simulink model "sampleModel386_pp_100_1"  (R2021b)
settings: Solver=VariableStepAuto  StartTime=0.0  StopTime=10.0  RelTol=1e-3
libraries: simulink x2, slpidlib x1
settings Model: Creator=user  LastModifiedBy=cemery

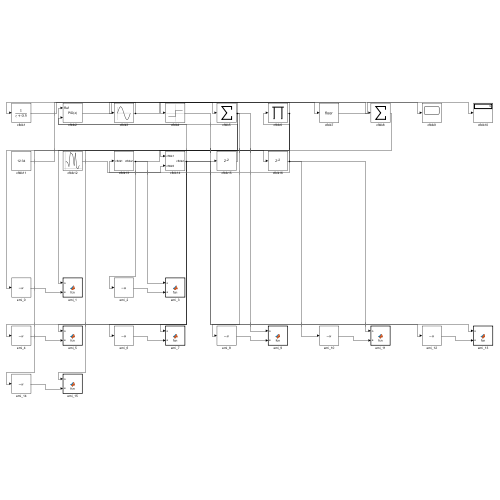
[thumbnail: Simulink's stored preview of the top-level diagram]
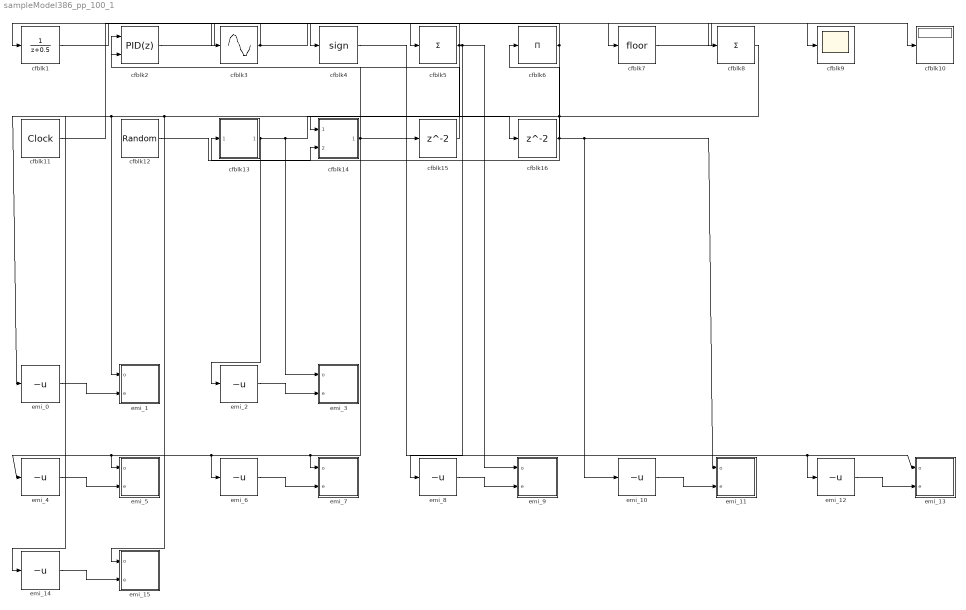
== system sampleModel386_pp_100_1 ==
  cfblk1 : DiscreteTransferFcn  SampleTime=1
  cfblk10 : Display
  cfblk11 : DigitalClock
  cfblk12 : RandomNumber  Mean=[-91757.722455]  Variance=[72797.748445]  Seed=[931341017.000000]  SampleTime=0.1
  cfblk13 : Subsystem
  cfblk14 : Subsystem
  cfblk15 : Delay  SampleTime=1
  cfblk16 : Delay  SampleTime=1
  cfblk2 : slpidlib/PID Controller (2DOF)  Controller=PID  Form=Parallel  TimeDomain=Discrete-time  UseExternalTs=off  SampleTime=1  IntegratorMethod=Forward Euler  FilterMethod=Forward Euler  ControllerParametersSource=internal  P=1  I=1  D=0  UseFilter=on  N=100  b=1  c=1  TunerSelectOption=Transfer Function Based (PID Tuner App)  InitialConditionSource=internal  InitialConditionForIntegrator=0  InitialConditionForFilter=0  DifferentiatorICPrevScaledInput=0  ExternalReset=none  TrackingMode=off  Kt=1  LimitOutput=off  SatLimitsSource=internal  UpperSaturationLimit=inf  LowerSaturationLimit=-inf  LinearizeAsGain=off  AntiWindupMode=none  Kb=1  POutMin=[]  POutMax=[]  IOutMin=[]  IOutMax=[]  DOutMin=[]  DOutMax=[]  NOutMin=[]  NOutMax=[]  bOutMin=[]  bOutMax=[]  cOutMin=[]  cOutMax=[]  SumOutMin=[]  SumOutMax=[]  SaturationOutMin=[]  SaturationOutMax=[]  PParamMin=[]  PParamMax=[]  IParamMin=[]  IParamMax=[]  DParamMin=[]  DParamMax=[]  NParamMin=[]  NParamMax=[]  bParamMin=[]  bParamMax=[]  cParamMin=[]  cParamMax=[]  KbParamMin=[]  KbParamMax=[]  KtParamMin=[]  KtParamMax=[]  KbOutMin=[]  KbOutMax=[]  KtOutMin=[]  KtOutMax=[]  IntegratorOutMin=[]  IntegratorOutMax=[]  FilterOutMin=[]  FilterOutMax=[]  SumI1OutMin=[]  SumI1OutMax=[]  SumI2OutMin=[]  SumI2OutMax=[]  SumI3OutMin=[]  SumI3OutMax=[]  SumI4OutMin=[]  SumI4OutMax=[]  SumDOutMin=[]  SumDOutMax=[]  Sum1OutMin=[]  Sum1OutMax=[]  Sum2OutMin=[]  Sum2OutMax=[]  Sum3OutMin=[]  Sum3OutMax=[]  DifferentiatorOutMin=[]  DifferentiatorOutMax=[]  FilterDiffOutCoefMin=[]  FilterDiffOutCoefMax=[]  ReciprocalOutMin=[]  ReciprocalOutMax=[]  SumDenOutMin=[]  SumDenOutMax=[]  SumNumOutMin=[]  SumNumOutMax=[]  DivideOutMin=[]  DivideOutMax=[]  UdiffTsProdOutMin=[]  UdiffTsProdOutMax=[]  NTsProdOutMin=[]  NTsProdOutMax=[]  UintegralTsProdOutMin=[]  UintegralTsProdOutMax=[]  UngainTsProdOutMin=[]  UngainTsProdOutMax=[]  IntegratorContinuousStateAttributes=''  IntegratorStateMustResolveToSignalObject=off  IntegratorRTWStateStorageClass=Auto  FilterContinuousStateAttributes=''  FilterStateMustResolveToSignalObject=off  FilterRTWStateStorageClass=Auto  ParallelPVariant=InternalParameters  IdealPVariant=Disabled  IVariant=InternalParameters  DVariant=InternalParameters  bVariant=InternalParameters  cVariant=InternalParameters  IntegratorVariant=Discrete  SatVariant=Disabled  AWVariant=Passthrough  PCopyVariant=Disabled  TRVariant=Disabled  FdbkBlocksVariant=Forward  IdealPFdbkVariant=Disabled  SatFdbkVariant=Disabled  DerivativeFilterVariant=ForwardEulerFilter  NVariant=InternalParameters  NCopyVariant=Disabled  FilterICVariant=InternalICsFilter  IntegratorICVariant=InternalICs  ExternalResetVariant=Disabled  TRSumVariant=Passthrough  SumFdbkVariant=Disabled  SumVariant=Sum_PID  TsampFilterVariant=InternalTs  TsampNgainVariant=Passthrough  TsampIntegralVariant=Passthrough  ExternalSaturationOutDataTypeStr=Inherit: Same as second input
      settings: SourceProductBaseCode=SL
  cfblk3 : Sin  TimeSource=Use external signal  SampleTime=0
  cfblk4 : Signum
  cfblk5 : Sum  Inputs=+  OutDataTypeStr=double
  cfblk6 : Product  Inputs=*  OutDataTypeStr=double
  cfblk7 : Rounding
  cfblk8 : Sum  Inputs=+  OutDataTypeStr=double
  cfblk9 : Scope
  emi_{0,2,4,6,8,10,12,14} (8 alike) : UnaryMinus
  emi_1 : MATLAB Function  TreatAsAtomicUnit=on
  emi_11 : MATLAB Function  TreatAsAtomicUnit=on
  emi_13 : MATLAB Function  TreatAsAtomicUnit=on
  emi_15 : MATLAB Function  TreatAsAtomicUnit=on
  emi_3 : MATLAB Function  TreatAsAtomicUnit=on
  emi_5 : MATLAB Function  TreatAsAtomicUnit=on
  emi_7 : MATLAB Function  TreatAsAtomicUnit=on
  emi_9 : MATLAB Function  TreatAsAtomicUnit=on
  wires:
  cfblk14/1(cfblk2) -> emi_4/1, emi_5/1(o), emi_6/1, emi_7/1(o), emi_12/1, emi_13/1(o), cfblk2/1
  cfblk7/1 -> cfblk9/1
  cfblk6/1 -> emi_14/1, emi_15/1(o), cfblk13/1(cfblk1), cfblk3/1
  cfblk11/1 -> cfblk8/1
  cfblk8/1 -> cfblk14/1(cfblk1)
  cfblk5/1 -> emi_0/1, emi_1/1(o), emi_8/1, emi_9/1(o), cfblk4/1
  cfblk2/1 -> cfblk5/1
  cfblk1/1 -> cfblk7/1
  cfblk12/1 -> cfblk14/2(cfblk5)
  cfblk3/1 -> cfblk1/1, cfblk10/1
  cfblk4/1 -> cfblk15/1
  cfblk15/1 -> cfblk2/2
  cfblk13/1(cfblk2) -> cfblk16/1, emi_3/1(o), emi_2/1
  cfblk16/1 -> emi_10/1, emi_11/1(o), cfblk6/1
  emi_0/1 -> emi_1/2(e)
  emi_2/1 -> emi_3/2(e)
  emi_4/1 -> emi_5/2(e)
  emi_6/1 -> emi_7/2(e)
  emi_8/1 -> emi_9/2(e)
  emi_10/1 -> emi_11/2(e)
  emi_12/1 -> emi_13/2(e)
  emi_14/1 -> emi_15/2(e)

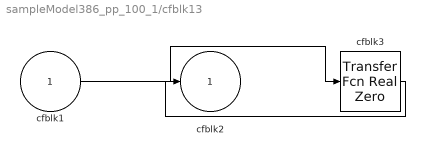
== system sampleModel386_pp_100_1/cfblk13 ==
  cfblk1 : Inport
  cfblk3 : simulink/Discrete/Transfer Fcn Real Zero  ZeroZ=0.75  ICPrevInput=0.0  DoSatur=off
      settings: SourceProductBaseCode=SL
  cfblk2 : Outport
  wires:
  cfblk1/1 -> cfblk3/1
  cfblk3/1 -> cfblk2/1

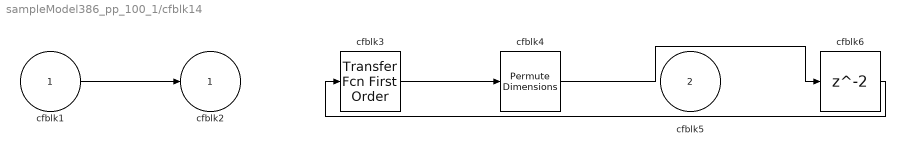
== system sampleModel386_pp_100_1/cfblk14 ==
  cfblk1 : Inport
  cfblk5 : Inport  Port=2
  cfblk3 : simulink/Discrete/Transfer Fcn First Order  PoleZ=0.95  ICPrevOutput=0.0  DoSatur=off
  cfblk4 : PermuteDimensions
  cfblk6 : Delay  SampleTime=1
  cfblk2 : Outport
  wires:
  cfblk1/1 -> cfblk2/1
  cfblk3/1 -> cfblk4/1
  cfblk4/1 -> cfblk6/1
  cfblk6/1 -> cfblk3/1

== matlab function sampleModel386_pp_100_1/emi_1 ==
  data: o input; e input
function  fcn(o, e)
o_inv = o^-1;
e_inv = e^-1;

emsg = 'sampleModel386_pp_100_1/emi_1';
 
if(o == e)
    assert(o_inv == e_inv, [emsg ' ; o_inv~=e_inv']);
    return;
end
 
if(o_inv > 0)
    assert(e_inv < 0, [emsg ' ; e_inv>=0']);
else
    assert(e_inv > 0, [emsg ' ; e_inv<=0']);
end

== matlab function sampleModel386_pp_100_1/emi_5 ==
  data: o input; e input
function  fcn(o, e)
o_inv = o^-1;
e_inv = e^-1;

emsg = 'sampleModel386_pp_100_1/emi_5';
 
if(o == e)
    assert(o_inv == e_inv, [emsg ' ; o_inv~=e_inv']);
    return;
end
 
if(o_inv > 0)
    assert(e_inv < 0, [emsg ' ; e_inv>=0']);
else
    assert(e_inv > 0, [emsg ' ; e_inv<=0']);
end

== matlab function sampleModel386_pp_100_1/emi_7 ==
  data: o input; e input
function  fcn(o, e)
o_inv = o^-1;
e_inv = e^-1;

emsg = 'sampleModel386_pp_100_1/emi_7';
 
if(o == e)
    assert(o_inv == e_inv, [emsg ' ; o_inv~=e_inv']);
    return;
end
 
if(o_inv > 0)
    assert(e_inv < 0, [emsg ' ; e_inv>=0']);
else
    assert(e_inv > 0, [emsg ' ; e_inv<=0']);
end

== matlab function sampleModel386_pp_100_1/emi_9 ==
  data: o input; e input
function  fcn(o, e)
o_inv = o^-1;
e_inv = e^-1;

emsg = 'sampleModel386_pp_100_1/emi_9';
 
if(o == e)
    assert(o_inv == e_inv, [emsg ' ; o_inv~=e_inv']);
    return;
end
 
if(o_inv > 0)
    assert(e_inv < 0, [emsg ' ; e_inv>=0']);
else
    assert(e_inv > 0, [emsg ' ; e_inv<=0']);
end

== matlab function sampleModel386_pp_100_1/emi_11 ==
  data: o input; e input
function  fcn(o, e)
o_inv = o^-1;
e_inv = e^-1;

emsg = 'sampleModel386_pp_100_1/emi_11';
 
if(o == e)
    assert(o_inv == e_inv, [emsg ' ; o_inv~=e_inv']);
    return;
end
 
if(o_inv > 0)
    assert(e_inv < 0, [emsg ' ; e_inv>=0']);
else
    assert(e_inv > 0, [emsg ' ; e_inv<=0']);
end

== matlab function sampleModel386_pp_100_1/emi_13 ==
  data: o input; e input
function  fcn(o, e)
o_inv = o^-1;
e_inv = e^-1;

emsg = 'sampleModel386_pp_100_1/emi_13';
 
if(o == e)
    assert(o_inv == e_inv, [emsg ' ; o_inv~=e_inv']);
    return;
end
 
if(o_inv > 0)
    assert(e_inv < 0, [emsg ' ; e_inv>=0']);
else
    assert(e_inv > 0, [emsg ' ; e_inv<=0']);
end

== matlab function sampleModel386_pp_100_1/emi_15 ==
  data: o input; e input
function  fcn(o, e)
o_inv = o^-1;
e_inv = e^-1;

emsg = 'sampleModel386_pp_100_1/emi_15';
 
if(o == e)
    assert(o_inv == e_inv, [emsg ' ; o_inv~=e_inv']);
    return;
end
 
if(o_inv > 0)
    assert(e_inv < 0, [emsg ' ; e_inv>=0']);
else
    assert(e_inv > 0, [emsg ' ; e_inv<=0']);
end

== matlab function sampleModel386_pp_100_1/emi_3 ==
  data: o input; e input
function  fcn(o, e)
o_inv = o^-1;
e_inv = e^-1;

emsg = 'sampleModel386_pp_100_1/emi_3';
 
if(o == e)
    assert(o_inv == e_inv, [emsg ' ; o_inv~=e_inv']);
    return;
end
 
if(o_inv > 0)
    assert(e_inv < 0, [emsg ' ; e_inv>=0']);
else
    assert(e_inv > 0, [emsg ' ; e_inv<=0']);
end
